simulink model "Kart"  (R2026a)
settings: Solver=ode45  StopTime=40  EnableMultiTasking=on
values from neighbouring files (symbols this model uses):
  AD = 0.5*A*Cd*p    (= 0.1803)    [Kartdata.m]    (also in kartdata.m)
  FD = Mass*g*RRc    (= 39.24)    [Kartdata.m]    (also in kartdata.m)
  Gr = 2    [Kartdata.m]    (also in kartdata.m)
  KT = 0.12    [DCmototdata.m]    (also in Kartdata.m; dc_motor_data.m; kartdata.m)
  KV = 0.127    [DCmototdata.m]    (also in Kartdata.m; dc_motor_data.m; kartdata.m)
  La = 0.01    [DCmototdata.m]    (also in Kartdata.m; dc_motor_data.m; kartdata.m)
  Mass = 200    [Kartdata.m]    (also in kartdata.m)
  Ra = 0.053    [DCmototdata.m]    (also in Kartdata.m; dc_motor_data.m; kartdata.m)
  Rw = .125    (= 0.125)    [Kartdata.m]    (also in kartdata.m)
  vt = [34.6410161514 33.1662479036 31.6227766017 30 28.2842712475 26.4575131106 24.4948974278 22.360679775 20 17.3205080757 14.1421356237 14.1421356237 ... (48 elements, 1x48)]    [xt.mat]
  xt = [0 10 20 30 40 50 60 70 80 90 100 179 ... (48 elements, 1x48)]    [xt.mat]
libraries: sl_discontinuities x1
settings Model: Creator=Bob  LastModifiedBy=suria
settings SolverCC: ZeroCrossControl=DisableAll
settings DataIOCC: SaveFormat=StructureWithTime  SignalLoggingSaveFormat=ModelDataLogs
settings DebuggingCC: UnderspecifiedInitializationDetection=Classic
settings HardwareCC: ProdHWDeviceType=32-bit Generic
settings GRTTargetCC: CombineOutputUpdateFcns=off  GRTInterface=on

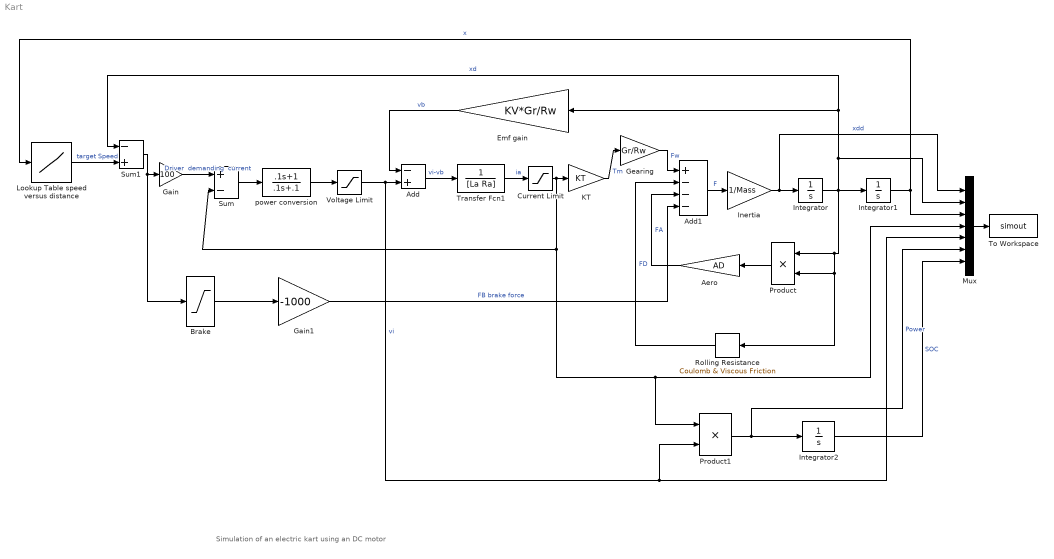
== system Kart ==
  note: Simulation of an electric kart using an DC motor
  Add : Sum  Inputs=-+
  Add1 : Sum  Inputs=+---
  Aero : Gain  Gain=AD
  Brake : Saturate  UpperLimit=0  LowerLimit=-1000
  Current Limit : Saturate  UpperLimit=300  LowerLimit=0
  Emf gain : Gain  Gain=KV*Gr/Rw
  Gain : Gain  Gain=100
  Gain1 : Gain  Gain=-1000
  Gearing : Gain  Gain=Gr/Rw
  Inertia : Gain  Gain=1/Mass
  Integrator : Integrator
  Integrator1 : Integrator
  Integrator2 : Integrator
  KT : Gain  Gain=KT
  Lookup Table speed versus distance : Lookup  InputValues=xt  Table=vt  SaturateOnIntegerOverflow=off
  Mux : Mux  Inputs=7
  Product : Product  RndMeth=Zero
  Product1 : Product  RndMeth=Zero
  Rolling Resistance : sl_discontinuities/Coulomb & Viscous Friction  offset=[FD]  gain=0
  Sum : Sum  Inputs=+-
  Sum1 : Sum  Inputs=-+
  To Workspace : ToWorkspace  VariableName=simout  SaveFormat=Structure  SampleTime=-1
  Transfer Fcn1 : TransferFcn  Denominator=[La Ra]
  Voltage Limit : Saturate  UpperLimit=48  LowerLimit=0
  power conversion : TransferFcn  Numerator=[.1 1]  Denominator=[.1 .1]
  wires:
  Add1/1 -> Inertia/1  "F"
  Gearing/1 -> Add1/1  "Fw"
  Add/1 -> Transfer Fcn1/1  "vi-vb"
  Emf gain/1 -> Add/1  "vb"
  Product/1 -> Aero/1
  Aero/1 -> Add1/3  "FA"
  Integrator/1 -> Mux/2, Emf gain/1, Sum1/1, Product/1, Product/2, Rolling Resistance/1, Integrator1/1  "xd"
  Integrator1/1 -> Mux/3, Lookup Table speed versus distance/1  "x"
  Mux/1 -> To Workspace/1
  Voltage Limit/1 -> Add/2, Mux/5, Product1/2  "vi"
  Product1/1 -> Integrator2/1, Mux/6  "Power"
  power conversion/1 -> Voltage Limit/1
  Integrator2/1 -> Mux/7  "SOC"
  Sum/1 -> power conversion/1
  Lookup Table speed versus distance/1 -> Sum1/2  "target Speed"
  Gain/1 -> Sum/1  "Driver  demanding  current"
  Sum1/1 -> Gain/1, Brake/1
  Transfer Fcn1/1 -> Current Limit/1  "ia"
  Current Limit/1 -> Sum/2, Mux/4, Product1/1, KT/1
  KT/1 -> Gearing/1  "Tm"
  Inertia/1 -> Integrator/1, Mux/1  "xdd"
  Brake/1 -> Gain1/1
  Gain1/1 -> Add1/4  "FB brake force"
  Rolling Resistance/1 -> Add1/2  "FD"
